simulink model "CSRT_Linear"  (R2020b)
settings: Solver=FixedStepAuto  StartTime=0.0  StopTime=15  FixedStep=0.01  RelTol=1e-3
values from neighbouring files (symbols this model uses):
  A = [A11, A12; A21, A22]    [Exp2_CSRT.m]
  B = horzcat(Bu, Bd)    [Exp2_CSRT.m]
  C = [1, 0]    [Exp2_CSRT.m]
  Cas = 8.564    [Exp2_CSRT.m]
  D = [0, 0, 0, 0]    [Exp2_CSRT.m]
settings Model: Creator=franc  LastModifiedBy=franc

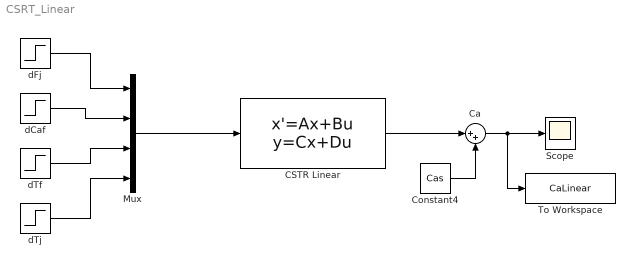
== system CSRT_Linear ==
  "              Ca" : Sum  Inputs=|++
  CSTR Linear : StateSpace  A=A  B=B  C=C  D=D  InitialCondition=0
  Constant4 : Constant  Value=Cas
  Mux : Mux
  Scope : Scope
  To Workspace : ToWorkspace  VariableName=CaLinear  SaveFormat=Timeseries  SampleTime=-1
  dCaf : Step  Time=0  After=0  SampleTime=0
  dFj : Step  Time=0  After=0.01  SampleTime=0
  dTf : Step  Time=0  After=0  SampleTime=0
  dTj : Step  Time=0  After=0  SampleTime=0
  wires:
  Mux/1 -> CSTR Linear/1
  dFj/1 -> Mux/1
  dCaf/1 -> Mux/2
  dTf/1 -> Mux/3
  dTj/1 -> Mux/4
  CSTR Linear/1 -> "              Ca"/1
  Constant4/1 -> "              Ca"/2
  "              Ca"/1 -> To Workspace/1, Scope/1
